simulink model "Programmer_Calculator"  (R2016a)
settings: Solver=FixedStepDiscrete  StartTime=0.0  StopTime=10.0  RelTol=1e-3
settings Model: Creator=NoteBook  LastModifiedBy=NoteBook
settings OptimizationCC: DefaultParameterBehavior=Inlined  EnableMemcpy=off  OptimizeModelRefInitCode=on  LifeSpan=1
settings DebuggingCC: UnderspecifiedInitializationDetection=Classic  MergeDetectMultiDrivingBlocksExec=none
settings ModelReferenceCC: PropagateSignalLabelsOutOfModel=off
settings RTWCC: SystemTargetFile=ert.tlc  GenCodeOnly=on  TemplateMakefile=ert_default_tmf  GenerateReport=on  IncludeHyperlinkInReport=on  LaunchReport=on  GenerateTraceInfo=on  GenerateTraceReport=on  GenerateTraceReportSl=on  GenerateTraceReportSf=on  GenerateTraceReportEml=on
settings CodeAppCC: ForceParamTrailComments=on  IgnoreCustomStorageClasses=off  OperatorAnnotations=on  SimulinkDataObjDesc=on  SFDataObjDesc=on  MATLABFcnDesc=on  InsertBlockDesc=on  MATLABSourceComments=on
settings ERTTargetCC: GenerateSampleERTMain=on  InlinedParameterPlacement=NonHierarchical  ERTCustomFileTemplate=example_file_process.tlc

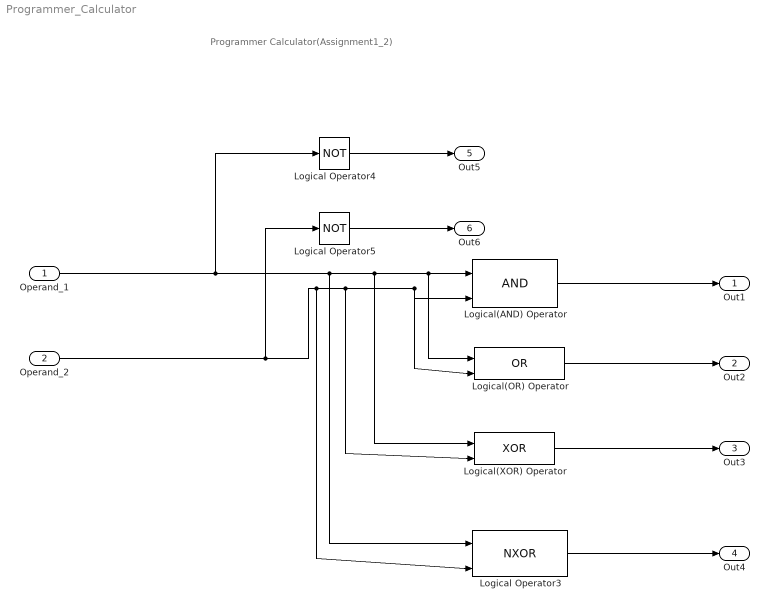
== system Programmer_Calculator ==
  note: Programmer Calculator(Assignment1_2)
  "Operand_1 " : Inport  OutDataTypeStr=uint8
  Operand_2 : Inport  Port=2  OutDataTypeStr=uint8
  Logical Operator3 : Logic  Operator=NXOR  IconShape=distinctive  AllPortsSameDT=off
  Logical Operator4 : Logic  Operator=NOT  IconShape=distinctive  AllPortsSameDT=off
  Logical Operator5 : Logic  Operator=NOT  Inputs=1  IconShape=distinctive  AllPortsSameDT=off
  Logical(AND) Operator : Logic  IconShape=distinctive  AllPortsSameDT=off
  "Logical(OR) Operator " : Logic  Operator=OR  IconShape=distinctive  AllPortsSameDT=off
  "Logical(XOR) Operator " : Logic  Operator=XOR  IconShape=distinctive  AllPortsSameDT=off
  Out1 : Outport
  Out2 : Outport  Port=2
  Out3 : Outport  Port=3
  Out4 : Outport  Port=4
  Out5 : Outport  Port=5
  Out6 : Outport  Port=6
  wires:
  "Operand_1 "/1 -> Logical Operator4/1, Logical Operator3/1, "Logical(XOR) Operator "/1, "Logical(OR) Operator "/1, Logical(AND) Operator/1
  Operand_2/1 -> Logical Operator5/1, Logical Operator3/2, "Logical(XOR) Operator "/2, "Logical(OR) Operator "/2, Logical(AND) Operator/2
  Logical(AND) Operator/1 -> Out1/1
  Logical Operator4/1 -> Out5/1
  Logical Operator5/1 -> Out6/1
  "Logical(OR) Operator "/1 -> Out2/1
  "Logical(XOR) Operator "/1 -> Out3/1
  Logical Operator3/1 -> Out4/1
